simulink model "Feeder_IREQ_2012"  (Simulink 8.3)
settings: Solver=FixedStepDiscrete  StartTime=0.0  StopTime=100  FixedStep=50e-6  RelTol=1e-3
InitFcn:
  | Ts= 50e-6;
undefined symbols (not defined in the file): D11, Delta, DiscIntNeverNeededParam, Ion, kaimal_num, Lithium, u0
libraries: powerlib x62, powerlib_extras x49, simulink x14, simulink_extras x12, sps_avr x2, electricdrivelib x1
(part 2 of 5)

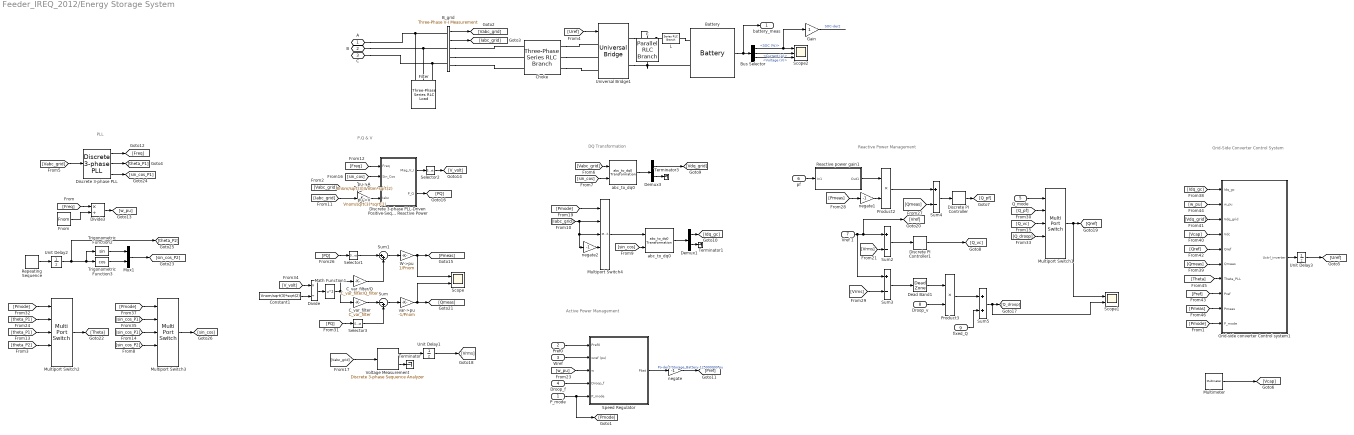
== system Feeder_IREQ_2012/Energy Storage System ==
  note: Grid-Side Converter
      | Control System
  note: DQ Transformation
  note: P,Q & V
  note: Reactive Power Management
  note: Active Power Management
  note: PLL
  P_mode : Inport
  Pref0 : Inport  Port=2
  Wref : Inport  Port=3
  Droop_f : Inport  Port=4
  Q_mode : Inport  Port=5
  "pf " : Inport  Port=6
  Vref 1 : Inport  Port=7
  Droop_v : Inport  Port=8
  fixed_Q : Inport  Port=9
  " C " : powerlib/Elements/Parallel RLC Branch  LConnTagsString=a  RConnTagsString=__new0  BranchType=C  Resistance=1  Inductance=1e-3  SetiL0=off  InitialCurrent=0  Capacitance=3000e-6  Setx0=on  InitialVoltage=Vbat  Measurements=Branch voltage
  B_grid : powerlib/Measurements/Three-Phase V-I Measurement  VoltageMeasurement=phase-to-ground  SetLabelV=off  LabelV=Vabc  Vpu=on  VpuLL=off  CurrentMeasurement=yes  SetLabelI=off  LabelI=Iabc  Ipu=on  Pbase=Pnom  Vbase=Vnom  OutputType=Complex  PhasorSimulation=off  PSBequivalent=0
  Battery : electricdrivelib/Extra Sources/Battery  BatType=Lithium-Ion  ShowDetailedParameters=off  NomV=Vbat  NomQ=Ebat/Vbat  SOC=SOC_initial  PresetModel=on  MaxQ=NaN  Dis_rate=NaN  Normal_OP=NaN  expZone="[NaN  NaN]"  Dis_Char=off  current=[1.5 3]  Units=Ampere-hour  Batt_Tr=10
  Bus Selector : BusSelector  OutputSignals=SOC (%),Current (A),Voltage (V)
  C_var_filter : Gain  Gain=C_var_filter  SaturateOnIntegerOverflow=on  OutDataTypeStr=Inherit: Same as input  ParamDataTypeStr=Inherit: Same as input
  C_var_filter/Q : Gain  Gain=C_var_filter/Q_filter  SaturateOnIntegerOverflow=on  OutDataTypeStr=Inherit: Same as input  ParamDataTypeStr=Inherit: Same as input
  "Choke " : powerlib/Elements/Three-Phase Series RLC Branch  LConnTagsString=A|B|C  RConnTagsString=A|B|C  BranchType=RL  Resistance=R_RL*Vnom^2/Pnom  Inductance=L_RL*Vnom^2/Pnom/(2*pi*Fnom)  Capacitance=[]  Measurements=None
  Constant1 : Constant  Value=Vnom/sqrt(3)*sqrt(2)
  Dead Band1 : DeadZone  LowerValue=-0.01  UpperValue=0.01  SaturateOnIntegerOverflow=on
  Demux1 : Demux  Outputs=[2 1]
  Demux3 : Demux  Outputs=[2 1]
  Discrete 3-phase PLL : powerlib_extras/Discrete  Control Blocks/Discrete 3-phase PLL  Fmin=0.75*Fnom  Par_Init=[-45 Fnom]  ParK=[60 1400 1]  Ts=Ts  AGC=off
  Discrete PI Controller : powerlib_extras/Discrete  Control Blocks/Discrete PI Controller  Kp=1  Ki=10  Par_Limits=[1 -1]  Init=0  Ts=-1
  Discrete PI Controller1 : powerlib_extras/Discrete  Control Blocks/Discrete PI Controller  Kp=2  Ki=20  Par_Limits=[1 -1]  Init=0  Ts=-1
  Discrete 3-phase PLL-Driven  Positive-Sequence Active & Reactive Power : Subsystem  mask(Discrete 3-phase PLL-Driven Positive-Sequence Active & Reactive Power){Finit=Fnom, Fmin=Fnom*45/60, Par_Vinit=[Vnom/sqrt(3)*sqrt(2) 30], Par_Iinit=[Pnom/sqrt(3)/Vnom*sqrt(2) -10], Ts=Ts}
      mask prompts: Finit "Initial frequency (Hz):"; Fmin "Minimum frequency (Hz):"; Par_Vinit "Voltage initial input: [ Mag  Phase(Degrees) ]"; Par_Iinit "Current initial input: [ Mag  Phase(Degrees) ]"; Ts "Sample time:"
      mask help:
      | This discrete block measures the 3-phase active power P and reactive power Q  associated with a periodic set of 3-phase voltages and currents which may contain harmonics. P and Q are calculated by evaluating the fundamental values (positive-sequence) of the input voltages and currents with a running window over one cycle of the specified frequency (port Freq).
      |  Input port "Sin_Cos" (a two-dimension signal) provides the reference frame required for the computation.
      |
      | input 1: must give the frequency of the fundamental (Hz)
      | Input 2: must contain a  [sin(wt)  cos(wt)] two dimension signal , where w is the rotation speed (rad/s) of the reference frame used for the computation..
      | input 3: Vectorized 3-phase  instantaneous voltage (Vabc)
      | input 4: Vectorized 3-phase instantaneous current (Iabc)
      |
      | Output 1: Vector [Mag_V Mag_I] of the fundamental values (Magnitude) of the voltage & current (peak values of the positive-sequence)
      | Output 2: 3-phase PQ measurement vector [P(W) Q (var)] evaluated at the specified frequency. Current flowing into an RL circuit will produce  positive active and reactive powers.
      |
      | For the first cycle of simulation, the outputs are held constant using the values specified by the parameters "Initial input".
      | he value of the parameter "Minimum frequency" is used to determine the buffer size of the "Variable Transport Delay" block found inside this subsystem.
      mask init:
      | power_initmask();
      settings: OpenFcn=power_openblockproxy();
  Divide : Product  Inputs=*/
  Divide3 : Product  Inputs=*/
  "Filter " : powerlib/Elements/Three-Phase Series RLC Load  LConnTagsString=A|B|C  Configuration=Y (grounded)  NominalVoltage=Vnom  NominalFrequency=Fnom  ActivePower=C_var_filter/Q_filter  InductivePower=0  CapacitivePower=C_var_filter  Measurements=None  LoadType=constant Z
  Fnom : Constant  Value=Fnom
  Gain : Gain
  Grid-side converter Control system1 : Subsystem
  L : powerlib/Elements/Series RLC Branch  LConnTagsString=__new0  RConnTagsString=__new0  BranchType=L  Resistance=1  Inductance=10e-6  SetiL0=off  InitialCurrent=0  Capacitance=1e-6  Setx0=off  InitialVoltage=0  Measurements=None
  Math Function1 : Math  Operator=square  SaturateOnIntegerOverflow=on
  Multimeter : powerlib/Measurements/Multimeter  PhasorSimulation=off  OutputType=Complex  sel=2  L=3  Gain=1  yselected={'Ub: Energy Storage System/ C '};  PSBOutputType=1  PSBequivalent=0  AxesSetting=[0,0.1,-100,100]  Display=0  SavedBlockNames=-11
  Multiport Switch{1..4} (4 alike) : MultiPortSwitch  Inputs=4  SaturateOnIntegerOverflow=on  InputSameDT=on
  Mux1 : Mux  Inputs=2
  Product2 : Product  RndMeth=Zero
  Product3 : Product  RndMeth=Zero
  Reactive power gain1 : Subsystem
  Repeating Sequence : simulink/Sources/Repeating Sequence  rep_seq_t=[0 1/60]  rep_seq_y=[0 2*pi]
  Scope : Scope  NumInputPorts=2
  Scope1 : Scope  NumInputPorts=2
  Scope2 : Scope  NumInputPorts=3
  Selector1 : Selector  InputPortWidth=2
  Selector2 : Selector  InputPortWidth=2
  Selector3 : Selector  InputPortWidth=2  Indices=2
  Speed Regulator : Subsystem  mask(Active Power Control){}
  Sum : Sum  Inputs=|-+
  Sum1 : Sum  Inputs=|++
  Sum2 : Sum  Inputs=+-  SaturateOnIntegerOverflow=on  InputSameDT=on  OutDataTypeStr=Inherit: Same as first input
  Sum3 : Sum  Inputs=+-  SaturateOnIntegerOverflow=on  InputSameDT=on  OutDataTypeStr=Inherit: Same as first input
  Sum4 : Sum  Inputs=+-  SaturateOnIntegerOverflow=on  InputSameDT=on  OutDataTypeStr=Inherit: Same as first input
  Sum5 : Sum  SaturateOnIntegerOverflow=on  InputSameDT=on  OutDataTypeStr=Inherit: Same as first input
  Terminator : Terminator
  Terminator1 : Terminator
  Terminator3 : Terminator
  Trigonometric Function2 : Trigonometry
  Trigonometric Function3 : Trigonometry  Operator=cos
  Unit Delay1 : UnitDelay  InitialCondition=1  SampleTime=Ts
  Unit Delay2 : UnitDelay  SampleTime=Ts
  Unit Delay3 : UnitDelay  SampleTime=Ts
  Universal Bridge1 : powerlib/Power Electronics/Universal Bridge  Arms=3  SnubberResistance=1e5  SnubberCapacitance=inf  Device=Average-model based VSC  Ron=1e-3  Lon=0  ForwardVoltages="[  0  0  ]"  ForwardVoltage=0  GTOparameters=[ 10e-6 , 20e-6 ]  IGBTparameters=[ 1e-6 , 2e-6 ]  Measurements=None  Measurements_2=None  converterType=Rectifier
  Voltage Measurement : powerlib_extras/Discrete Measurements/Discrete 3-phase Sequence Analyzer  Freq=60  n=1  seq=Positive  Par_Init=[1 0]  Ts=50e-6
  W->pu : Gain  Gain=1/Pnom  SaturateOnIntegerOverflow=on  OutDataTypeStr=Inherit: Same as input  ParamDataTypeStr=Inherit: Same as input
  abc_to_dq0 : powerlib_extras/Measurements/abc_to_dq0 Transformation
  "abc_to_dq0  " : powerlib_extras/Measurements/abc_to_dq0 Transformation
  negate : Gain  Gain=-1  SaturateOnIntegerOverflow=on  OutDataTypeStr=Inherit: Same as input  ParamDataTypeStr=Inherit: Same as input
  negate1 : Gain  Gain=-1  SaturateOnIntegerOverflow=on  OutDataTypeStr=Inherit: Same as input  ParamDataTypeStr=Inherit: Same as input
  negate2 : Gain  Gain=-1  SaturateOnIntegerOverflow=on  OutDataTypeStr=Inherit: Same as input  ParamDataTypeStr=Inherit: Same as input
  pu->A : Gain  Gain=Pnom/sqrt(3)/Vnom*sqrt(2)  SaturateOnIntegerOverflow=on  OutDataTypeStr=Inherit: Same as input  ParamDataTypeStr=Inherit: Same as input
  pu->V : Gain  Gain=Vnom/sqrt(3)*sqrt(2)  SaturateOnIntegerOverflow=on  OutDataTypeStr=Inherit: Same as input  ParamDataTypeStr=Inherit: Same as input
  "var->pu " : Gain  Gain=-1/Pnom  SaturateOnIntegerOverflow=on  OutDataTypeStr=Inherit: Same as input  ParamDataTypeStr=Inherit: Same as input
  A : PMIOPort  Port=1  Side=Right
  B : PMIOPort  Port=2  Side=Right
  C : PMIOPort  Port=3  Side=Right
  battery_meas : Outport
  wires:
  Grid-side converter Control system1/1(Uctrl_inverter) -> Unit Delay3/1
  Fnom/1 -> Divide3/2
  Divide3/1 -> [w_pu]
  [Freq] -> Divide3/1
  Demux1/2 -> Terminator1/1
  Demux3/2 -> Terminator3/1
  "abc_to_dq0  "/1 -> Demux1/1
  abc_to_dq0/1 -> Demux3/1
  [Vabc_grid] -> abc_to_dq0/1
  [sin_cos] -> abc_to_dq0/2
  [sin_cos] -> "abc_to_dq0  "/2
  B_grid/1 -> [Vabc_grid]
  B_grid/2 -> [Iabc_grid]
  Unit Delay3/1 -> [Uref]
  Selector2/1 -> [V_volt]
  Discrete 3-phase PLL-Driven  Positive-Sequence Active & Reactive Power/1(Mag_V_I) -> Selector2/1
  pu->V/1 -> Discrete 3-phase PLL-Driven  Positive-Sequence Active & Reactive Power/3(Vabc)
  [Freq] -> Discrete 3-phase PLL-Driven  Positive-Sequence Active & Reactive Power/1(Freq)
  [sin_cos] -> Discrete 3-phase PLL-Driven  Positive-Sequence Active & Reactive Power/2(Sin_Cos)
  pu->A/1 -> Discrete 3-phase PLL-Driven  Positive-Sequence Active & Reactive Power/4(Iabc)
  [Vabc_grid] -> pu->V/1
  [Iabc_grid] -> pu->A/1
  Discrete 3-phase PLL-Driven  Positive-Sequence Active & Reactive Power/2(P_Q) -> [PQ]
  "var->pu "/1 -> [Qmeas], Scope/2
  [PQ] -> Selector3/1
  W->pu/1 -> [Pmeas], Scope/1
  [PQ] -> Selector1/1
  [V_volt] -> Divide/1
  Constant1/1 -> Divide/2
  Divide/1 -> Math Function1/1
  Selector3/1 -> Sum/2
  Sum/1 -> "var->pu "/1
  Math Function1/1 -> C_var_filter/Q/1, C_var_filter/1
  Selector1/1 -> Sum1/1
  Sum1/1 -> W->pu/1
  [Uref] -> Universal Bridge1/1
  [Qmeas] -> Sum4/2
  Sum4/1 -> Discrete PI Controller/1
  [Pmeas] -> negate1/1
  Vref 1/1 -> [Vref], Sum2/1, Sum3/1
  [Vrms] -> Sum2/2
  Sum2/1 -> Discrete PI Controller1/1
  Reactive power gain1/1(Out1) -> Product2/1
  Product2/1 -> Sum4/1
  [Vrms] -> Sum3/2
  Sum3/1 -> Dead Band1/1
  Discrete PI Controller/1 -> [Q_pf]
  Dead Band1/1 -> Product3/1
  Droop_v/1 -> Product3/2
  Product3/1 -> Sum5/1
  Sum5/1 -> Scope1/2, [Q_droop]
  fixed_Q/1 -> Sum5/2
  [Q_pf] -> Multiport Switch1/2
  [Q_vc] -> Multiport Switch1/3
  [Q_droop] -> Multiport Switch1/4
  Q_mode/1 -> Multiport Switch1/1
  [Vabc_grid] -> Voltage Measurement/1
  Voltage Measurement/2 -> Terminator/1
  Voltage Measurement/1 -> Unit Delay1/1
  Unit Delay1/1 -> [Vrms]
  Pref0/1 -> Speed Regulator/1(Pref0)
  Wref/1 -> Speed Regulator/2(wref (pu))
  [w_pu] -> Speed Regulator/3(w)
  Droop_f/1 -> Speed Regulator/4(Droop_f)
  P_mode/1 -> Speed Regulator/5(P_mode), [Pmode]
  Speed Regulator/1(Pbat) -> negate/1
  Multiport Switch1/1 -> Scope1/1, [Qref]
  negate1/1 -> Product2/2
  "pf "/1 -> Reactive power gain1/1(In1)
  Multimeter/1 -> [Vcap]
  Trigonometric Function3/1 -> Mux1/2
  Trigonometric Function2/1 -> Mux1/1
  Unit Delay2/1 -> [theta_P2], Trigonometric Function2/1, Trigonometric Function3/1
  [Vabc_grid] -> Discrete 3-phase PLL/1
  Discrete 3-phase PLL/1 -> [Freq]
  Discrete 3-phase PLL/2 -> [theta_P1]
  Discrete 3-phase PLL/3 -> [sin_cos_P1]
  Mux1/1 -> [sin_cos_P2]
  [theta_P1] -> Multiport Switch2/2
  [Pmode] -> Multiport Switch2/1
  [sin_cos_P1] -> Multiport Switch3/2
  [Pmode] -> Multiport Switch3/1
  Multiport Switch2/1 -> [Theta]
  Multiport Switch3/1 -> [sin_cos]
  Discrete PI Controller1/1 -> [Q_vc]
  Repeating Sequence/1 -> Unit Delay2/1
  Demux3/1 -> [Vdq_grid]
  Demux1/1 -> [Idq_gc]
  [Idq_gc] -> Grid-side converter Control system1/1(Idq_gc)
  [w_pu] -> Grid-side converter Control system1/2(w_pu)
  [Vdq_grid] -> Grid-side converter Control system1/3(Vdq_grid)
  [Vcap] -> Grid-side converter Control system1/4(Vdc)
  [Qref] -> Grid-side converter Control system1/5(Qref)
  [Qmeas] -> Grid-side converter Control system1/6(Qmeas)
  [Theta] -> Grid-side converter Control system1/7(Theta_PLL)
  [Pref] -> Grid-side converter Control system1/8(Pref)
  [Pmeas] -> Grid-side converter Control system1/9(Pmeas)
  [Pmode] -> Grid-side converter Control system1/10(P_mode)
  [theta_P2] -> Multiport Switch2/4
  [sin_cos_P2] -> Multiport Switch3/4
  negate/1 -> [Pref]  "Po-der2-Storage_Battery-125000000-pu"
  [Pmode] -> Multiport Switch4/1
  [Iabc_grid] -> negate2/1, Multiport Switch4/3, Multiport Switch4/2
  negate2/1 -> Multiport Switch4/4
  Multiport Switch4/1 -> "abc_to_dq0  "/1
  C_var_filter/Q/1 -> Sum1/2
  C_var_filter/1 -> Sum/1
  [theta_P1] -> Multiport Switch2/3
  [sin_cos_P1] -> Multiport Switch3/3
  Battery/1 -> battery_meas/1, Bus Selector/1
  Bus Selector/2 -> Scope2/2  "<Current (A)>"
  Bus Selector/1 -> Gain/1, Scope2/1  "<SOC (%)>"
  Bus Selector/3 -> Scope2/3  "<Voltage (V)>"
  Gain/1 -> ?  "SOC-der2"
  connections:
  B_grid/RConn1 -- "Choke "/LConn1
  B_grid/RConn2 -- "Choke "/LConn2
  B_grid/RConn3 -- "Choke "/LConn3
  "Choke "/RConn1 -- Universal Bridge1/LConn1
  "Choke "/RConn2 -- Universal Bridge1/LConn2
  "Choke "/RConn3 -- Universal Bridge1/LConn3
  C/RConn1 -- "Filter "/LConn3 -- B_grid/LConn3
  B/RConn1 -- "Filter "/LConn2 -- B_grid/LConn2
  A/RConn1 -- B_grid/LConn1 -- "Filter "/LConn1
  L/LConn1 -- Universal Bridge1/RConn1 -- " C "/LConn1
  L/RConn1 -- Battery/LConn1
  Universal Bridge1/RConn2 -- " C "/RConn1 -- Battery/LConn2

== system Feeder_IREQ_2012/Kaimal Wind Speed Profile ==
  Band-Limited White Noise : simulink/Sources/Band-Limited White Noise  Cov=[1]  Ts=.05  seed=[53489]
  Constant4 : Constant  Value=Mean_wind
  Constant6 : Constant  Value=trans/sqrt(2)
  Product : Product  SampleTime=.05  RndMeth=Zero
  Rate Transition : RateTransition
  Sum1 : Sum  SampleTime=.05  SaturateOnIntegerOverflow=on  InputSameDT=on  OutDataTypeStr=Inherit: Same as first input
  Transfer Fcn Direct Form II : simulink/Additional Math & Discrete/Additional Discrete/Transfer Fcn Direct Form II  NumCoefVec=[kaimal_num]  DenCoefVec=[kaimal_den(2:end)]  vinit=0.0  DoSatur=off
  Unit Delay : UnitDelay  SampleTime=.05
  wind profile : Outport  InitialOutput=[u0]
  wires:
  Product/1 -> Sum1/2
  Constant6/1 -> Product/2
  Sum1/1 -> [wind], Rate Transition/1
  Constant4/1 -> Sum1/1
  Band-Limited White Noise/1 -> Unit Delay/1
  Transfer Fcn Direct Form II/1 -> Product/1
  Unit Delay/1 -> Transfer Fcn Direct Form II/1
  Rate Transition/1 -> wind profile/1

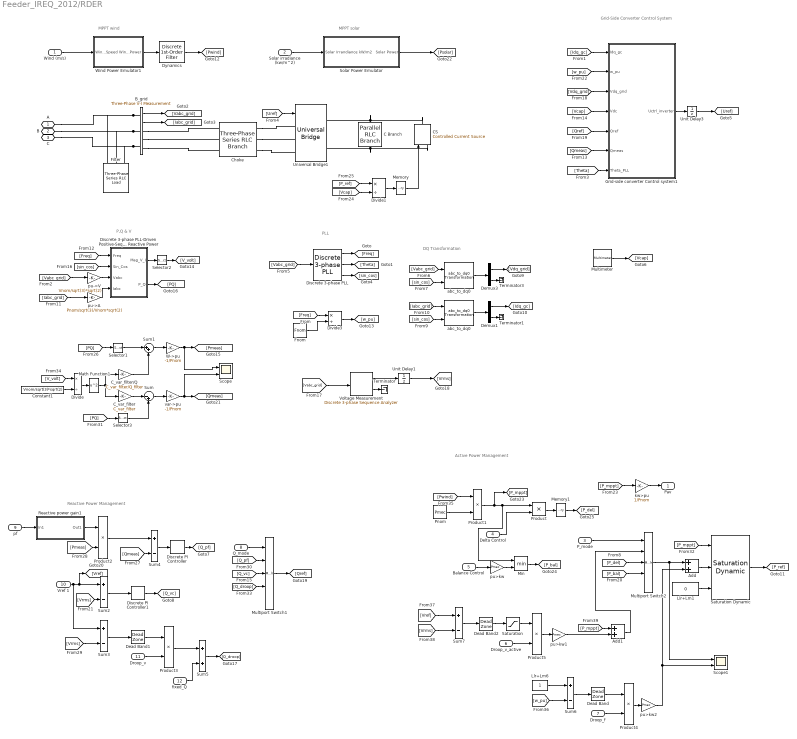
== system Feeder_IREQ_2012/RDER ==
  note: Grid-Side Converter
      | Control System
  note: PLL
  note: DQ Transformation
  note: P,Q & V
  note: Reactive Power Management
  note: Active Power Management
  note: MPPT wind
  note: MPPT solar
  "Wind (m/s) " : Inport
  Solar irradiance (kw/m^2) : Inport  Port=2
  P_mode : Inport  Port=3
  Delta Control : Inport  Port=4
  Balance Control : Inport  Port=5
  Droop_v_active : Inport  Port=6
  Droop_f : Inport  Port=7
  Q_mode : Inport  Port=8
  "pf " : Inport  Port=9
  Vref 1 : Inport  Port=10
  Droop_v : Inport  Port=11
  fixed_Q : Inport  Port=12
  " C Branch" : powerlib/Elements/Parallel RLC Branch  LConnTagsString=a  RConnTagsString=__new0  BranchType=C  Resistance=1  Inductance=1e-3  SetiL0=off  InitialCurrent=0  Capacitance=2000e-6  Setx0=on  InitialVoltage=Vdc_nom  Measurements=Branch voltage
  Add : Sum
  Add1 : Sum
  B_grid : powerlib/Measurements/Three-Phase V-I Measurement  VoltageMeasurement=phase-to-ground  SetLabelV=off  LabelV=Vabc  Vpu=on  VpuLL=off  CurrentMeasurement=yes  SetLabelI=off  LabelI=Iabc  Ipu=on  Pbase=Pnom  Vbase=Vnom  OutputType=Complex  PhasorSimulation=off  PSBequivalent=0
  CS : powerlib/Electrical Sources/Controlled Current Source  Initialize=on  Source_Type=AC  Amplitude=0  Phase=0  Frequency=0  Measurements=None
  C_var_filter : Gain  Gain=C_var_filter  SaturateOnIntegerOverflow=on  OutDataTypeStr=Inherit: Same as input  ParamDataTypeStr=Inherit: Same as input
  C_var_filter/Q : Gain  Gain=C_var_filter/Q_filter  SaturateOnIntegerOverflow=on  OutDataTypeStr=Inherit: Same as input  ParamDataTypeStr=Inherit: Same as input
  "Choke " : powerlib/Elements/Three-Phase Series RLC Branch  LConnTagsString=A|B|C  RConnTagsString=A|B|C  BranchType=RL  Resistance=R_RL*Vnom^2/Pnom  Inductance=L_RL*Vnom^2/Pnom/(2*pi*Fnom)  Capacitance=[]  Measurements=None
  Constant1 : Constant  Value=Vnom/sqrt(3)*sqrt(2)
  Dead Band : DeadZone  LowerValue=-0.001  UpperValue=0.001  SaturateOnIntegerOverflow=on
  Dead Band1 : DeadZone  LowerValue=-0.01  UpperValue=0.01  SaturateOnIntegerOverflow=on
  Dead Band2 : DeadZone  LowerValue=-0.01  UpperValue=0.01  SaturateOnIntegerOverflow=on
  Demux1 : Demux  Outputs=[2 1]
  Demux3 : Demux  Outputs=[2 1]
  Discrete 3-phase PLL : powerlib_extras/Discrete  Control Blocks/Discrete 3-phase PLL  Fmin=0.75*Fnom  Par_Init=[-45 Fnom]  ParK=[60 1400 1]  Ts=Ts  AGC=off
  Discrete PI Controller : powerlib_extras/Discrete  Control Blocks/Discrete PI Controller  Kp=1  Ki=10  Par_Limits=[1 -1]  Init=0  Ts=-1
  Discrete PI Controller1 : powerlib_extras/Discrete  Control Blocks/Discrete PI Controller  Kp=1  Ki=10  Par_Limits=[1 -1]  Init=0  Ts=-1
  Discrete 3-phase PLL-Driven  Positive-Sequence Active & Reactive Power : Subsystem  mask(Discrete 3-phase PLL-Driven Positive-Sequence Active & Reactive Power){Finit=Fnom, Fmin=Fnom*45/60, Par_Vinit=[Vnom/sqrt(3)*sqrt(2) 30], Par_Iinit=[Pnom/sqrt(3)/Vnom*sqrt(2) -10], Ts=Ts}
      mask prompts: Finit "Initial frequency (Hz):"; Fmin "Minimum frequency (Hz):"; Par_Vinit "Voltage initial input: [ Mag  Phase(Degrees) ]"; Par_Iinit "Current initial input: [ Mag  Phase(Degrees) ]"; Ts "Sample time:"
      mask help:
      | This discrete block measures the 3-phase active power P and reactive power Q  associated with a periodic set of 3-phase voltages and currents which may contain harmonics. P and Q are calculated by evaluating the fundamental values (positive-sequence) of the input voltages and currents with a running window over one cycle of the specified frequency (port Freq).
      |  Input port "Sin_Cos" (a two-dimension signal) provides the reference frame required for the computation.
      |
      | input 1: must give the frequency of the fundamental (Hz)
      | Input 2: must contain a  [sin(wt)  cos(wt)] two dimension signal , where w is the rotation speed (rad/s) of the reference frame used for the computation..
      | input 3: Vectorized 3-phase  instantaneous voltage (Vabc)
      | input 4: Vectorized 3-phase instantaneous current (Iabc)
      |
      | Output 1: Vector [Mag_V Mag_I] of the fundamental values (Magnitude) of the voltage & current (peak values of the positive-sequence)
      | Output 2: 3-phase PQ measurement vector [P(W) Q (var)] evaluated at the specified frequency. Current flowing into an RL circuit will produce  positive active and reactive powers.
      |
      | For the first cycle of simulation, the outputs are held constant using the values specified by the parameters "Initial input".
      | he value of the parameter "Minimum frequency" is used to determine the buffer size of the "Variable Transport Delay" block found inside this subsystem.
      mask init:
      | power_initmask();
      settings: OpenFcn=power_openblockproxy();
  Divide : Product  Inputs=*/
  Divide1 : Product  Inputs=*/
  Divide3 : Product  Inputs=*/
  Dynamics : powerlib_extras/Discrete  Control Blocks/Discrete 1st-Order Filter  FilterType=Lowpass  Tc=1/3  Ts=50e-6  Initialize=off  Vac_Init=[0.8 -25 60]  Vdc_Init=1  PlotResponse=off  param1=[1 500 0.1]
  "Filter " : powerlib/Elements/Three-Phase Series RLC Load  LConnTagsString=A|B|C  Configuration=Y (grounded)  NominalVoltage=Vnom  NominalFrequency=Fnom  ActivePower=C_var_filter/Q_filter  InductivePower=0  CapacitivePower=C_var_filter  Measurements=None  LoadType=constant Z
  Fnom : Constant  Value=Fnom
  Grid-side converter Control system1 : Subsystem
  Llr+Lm1 : Constant  Value=0
  Llr+Lm6 : Constant
  Math Function1 : Math  Operator=square  SaturateOnIntegerOverflow=on
  Memory : Memory  X0=100
  Memory1 : Memory  X0=.8
  Min : MinMax  Inputs=2
  Multimeter : powerlib/Measurements/Multimeter  PhasorSimulation=off  OutputType=Complex  sel=3  L=3  Gain=1  yselected={'Ub: RDER/ C Branch'};  PSBOutputType=1  PSBequivalent=0  AxesSetting=[0,0.1,-100,100]  Display=0  SavedBlockNames=-11
  Multiport Switch1 : MultiPortSwitch  Inputs=4  SaturateOnIntegerOverflow=on  InputSameDT=on
  Multiport Switch2 : MultiPortSwitch  Inputs=4  SaturateOnIntegerOverflow=on  InputSameDT=on
  Pnom : Constant  Value=Pmec
  Product{,1..5} (6 alike) : Product  RndMeth=Zero
  Reactive power gain1 : Subsystem
  Saturation : Saturate  UpperLimit=0  LowerLimit=-1
  Saturation Dynamic : simulink/Discontinuities/Saturation Dynamic  OutMin=[]  OutMax=[]  OutDataTypeStr=Inherit: Same as second input  OutDataType=fixdt(1, 16)  OutScaling=2^-10  DoSatur=off
  Scope : Scope  NumInputPorts=2
  Scope1 : Scope  NumInputPorts=2
  Selector1 : Selector  InputPortWidth=2
  Selector2 : Selector  InputPortWidth=2
  Selector3 : Selector  InputPortWidth=2  Indices=2
  Solar Power Emulator : Subsystem
  Sum : Sum  Inputs=|-+
  Sum1 : Sum  Inputs=|++
  Sum{2..4,6..7} (5 alike) : Sum  Inputs=+-  SaturateOnIntegerOverflow=on  InputSameDT=on  OutDataTypeStr=Inherit: Same as first input
  Sum5 : Sum  SaturateOnIntegerOverflow=on  InputSameDT=on  OutDataTypeStr=Inherit: Same as first input
  Terminator : Terminator
  Terminator1 : Terminator
  Terminator3 : Terminator
  Unit Delay1 : UnitDelay  InitialCondition=1  SampleTime=Ts
  Unit Delay3 : UnitDelay  SampleTime=Ts
  Universal Bridge1 : powerlib/Power Electronics/Universal Bridge  Arms=3  SnubberResistance=1e5  SnubberCapacitance=inf  Device=Average-model based VSC  Ron=1e-3  Lon=0  ForwardVoltages="[  0  0  ]"  ForwardVoltage=0  GTOparameters=[ 10e-6 , 20e-6 ]  IGBTparameters=[ 1e-6 , 2e-6 ]  Measurements=None  Measurements_2=None  converterType=Rectifier
  Voltage Measurement : powerlib_extras/Discrete Measurements/Discrete 3-phase Sequence Analyzer  Freq=60  n=1  seq=Positive  Par_Init=[1 0]  Ts=50e-6
  W->pu : Gain  Gain=-1/Pnom  SaturateOnIntegerOverflow=on  OutDataTypeStr=Inherit: Same as input  ParamDataTypeStr=Inherit: Same as input
  Wind Power Emulator1 : Subsystem
  abc_to_dq0 : powerlib_extras/Measurements/abc_to_dq0 Transformation
  "abc_to_dq0  " : powerlib_extras/Measurements/abc_to_dq0 Transformation
  kw>pu : Gain  Gain=1/Pnom
  pu->A : Gain  Gain=Pnom/sqrt(3)/Vnom*sqrt(2)  SaturateOnIntegerOverflow=on  OutDataTypeStr=Inherit: Same as input  ParamDataTypeStr=Inherit: Same as input
  pu->V : Gain  Gain=Vnom/sqrt(3)*sqrt(2)  SaturateOnIntegerOverflow=on  OutDataTypeStr=Inherit: Same as input  ParamDataTypeStr=Inherit: Same as input
  pu>kw : Gain  Gain=Pmec
  pu>kw1 : Gain  Gain=Pmec
  pu>kw2 : Gain  Gain=Pmec
  "var->pu " : Gain  Gain=-1/Pnom  SaturateOnIntegerOverflow=on  OutDataTypeStr=Inherit: Same as input  ParamDataTypeStr=Inherit: Same as input
  A : PMIOPort  Port=1  Side=Right
  B : PMIOPort  Port=2  Side=Right
  C : PMIOPort  Port=3  Side=Right
  Pav : Outport
  wires:
  [Idq_gc] -> Grid-side converter Control system1/1(Idq_gc)
  [w_pu] -> Grid-side converter Control system1/2(w_pu)
  [Vdq_grid] -> Grid-side converter Control system1/3(Vdq_grid)
  [Vcap] -> Grid-side converter Control system1/4(Vdc)
  [Qmeas] -> Grid-side converter Control system1/6(Qmeas)
  Grid-side converter Control system1/1(Uctrl_inverter) -> Unit Delay3/1
  Discrete 3-phase PLL/1 -> [Freq]
  Fnom/1 -> Divide3/2
  Divide3/1 -> [w_pu]
  Discrete 3-phase PLL/3 -> [sin_cos]
  [Freq] -> Divide3/1
  Discrete 3-phase PLL/2 -> [Theta]
  [Vabc_grid] -> Discrete 3-phase PLL/1
  Demux1/2 -> Terminator1/1
  Demux3/1 -> [Vdq_grid]
  Demux3/2 -> Terminator3/1
  "abc_to_dq0  "/1 -> Demux1/1
  abc_to_dq0/1 -> Demux3/1
  [Vabc_grid] -> abc_to_dq0/1
  [sin_cos] -> abc_to_dq0/2
  [sin_cos] -> "abc_to_dq0  "/2
  [Iabc_grid] -> "abc_to_dq0  "/1
  Demux1/1 -> [Idq_gc]
  B_grid/1 -> [Vabc_grid]
  B_grid/2 -> [Iabc_grid]
  Unit Delay3/1 -> [Uref]
  Selector2/1 -> [V_volt]
  Discrete 3-phase PLL-Driven  Positive-Sequence Active & Reactive Power/1(Mag_V_I) -> Selector2/1
  pu->V/1 -> Discrete 3-phase PLL-Driven  Positive-Sequence Active & Reactive Power/3(Vabc)
  [Freq] -> Discrete 3-phase PLL-Driven  Positive-Sequence Active & Reactive Power/1(Freq)
  [sin_cos] -> Discrete 3-phase PLL-Driven  Positive-Sequence Active & Reactive Power/2(Sin_Cos)
  pu->A/1 -> Discrete 3-phase PLL-Driven  Positive-Sequence Active & Reactive Power/4(Iabc)
  [Vabc_grid] -> pu->V/1
  [Iabc_grid] -> pu->A/1
  Discrete 3-phase PLL-Driven  Positive-Sequence Active & Reactive Power/2(P_Q) -> [PQ]
  "var->pu "/1 -> [Qmeas], Scope/2
  [PQ] -> Selector3/1
  W->pu/1 -> [Pmeas], Scope/1
  [PQ] -> Selector1/1
  [V_volt] -> Divide/1
  Constant1/1 -> Divide/2
  Divide/1 -> Math Function1/1
  Selector3/1 -> Sum/2
  Sum/1 -> "var->pu "/1
  Math Function1/1 -> C_var_filter/Q/1, C_var_filter/1
  Selector1/1 -> Sum1/1
  Sum1/1 -> W->pu/1
  [Uref] -> Universal Bridge1/1
  Multimeter/1 -> [Vcap]
  [Qmeas] -> Sum4/2
  Sum4/1 -> Discrete PI Controller/1
  [Pmeas] -> Product2/2
  Vref 1/1 -> [Vref], Sum2/1, Sum3/1
  [Vrms] -> Sum2/2
  Sum2/1 -> Discrete PI Controller1/1
  Reactive power gain1/1(Out1) -> Product2/1
  Product2/1 -> Sum4/1
  [Vrms] -> Sum3/2
  Sum3/1 -> Dead Band1/1
  Discrete PI Controller/1 -> [Q_pf]
  Discrete PI Controller1/1 -> [Q_vc]
  Dead Band1/1 -> Product3/1
  Droop_v/1 -> Product3/2
  Product3/1 -> Sum5/1
  Sum5/1 -> [Q_droop]
  fixed_Q/1 -> Sum5/2
  [Q_pf] -> Multiport Switch1/2
  [Q_vc] -> Multiport Switch1/3
  [Q_droop] -> Multiport Switch1/4
  Q_mode/1 -> Multiport Switch1/1
  [Vabc_grid] -> Voltage Measurement/1
  Voltage Measurement/2 -> Terminator/1
  Voltage Measurement/1 -> Unit Delay1/1
  Unit Delay1/1 -> [Vrms]
  Divide1/1 -> Memory/1
  [Vcap] -> Divide1/2
  [P_ref] -> Divide1/1
  Memory/1 -> CS/1
  "Wind (m/s) "/1 -> Wind Power Emulator1/1(Wind Speed)
  [Theta] -> Grid-side converter Control system1/7(Theta_PLL)
  [Qref] -> Grid-side converter Control system1/5(Qref)
  Pnom/1 -> Product1/2
  [Pwind] -> Product1/1
  Product1/1 -> [P_mppt], Min/1, Product/1
  Delta Control/1 -> Product/2
  kw>pu/1 -> Pav/1
  Balance Control/1 -> pu>kw/1
  pu>kw/1 -> Min/2
  Min/1 -> [P_bal]
  Product/1 -> Memory1/1
  Add1/1 -> Multiport Switch2/2
  [P_del] -> Multiport Switch2/3
  [P_bal] -> Multiport Switch2/4
  P_mode/1 -> Multiport Switch2/1
  Multiport Switch2/1 -> Scope1/1, Add/1
  Llr+Lm6/1 -> Sum6/1
  [w_pu] -> Sum6/2
  Sum6/1 -> Dead Band/1
  Dead Band/1 -> Product4/1
  Add/1 -> Saturation Dynamic/2
  Saturation Dynamic/1 -> [P_ref]
  [P_mppt] -> Saturation Dynamic/1
  Llr+Lm1/1 -> Saturation Dynamic/3
  Droop_f/1 -> Product4/2
  Product4/1 -> pu>kw2/1
  [Vref] -> Sum7/1
  [Vrms] -> Sum7/2
  Sum7/1 -> Dead Band2/1
  Dead Band2/1 -> Saturation/1
  Droop_v_active/1 -> Product5/2
  Product5/1 -> pu>kw1/1
  [P_mppt] -> Add1/1
  Saturation/1 -> Product5/1
  pu>kw1/1 -> Add1/2
  [P_mppt] -> kw>pu/1
  Dynamics/1 -> [Pwind]
  Solar Power Emulator/1(Solar Power) -> [Psolar]
  Wind Power Emulator1/1(Wind Power) -> Dynamics/1
  Solar irradiance (kw/m^2)/1 -> Solar Power Emulator/1(Solar Irrandiance kW/m2)
  C_var_filter/Q/1 -> Sum1/2
  C_var_filter/1 -> Sum/1
  Multiport Switch1/1 -> [Qref]
  "pf "/1 -> Reactive power gain1/1(In1)
  pu>kw2/1 -> Scope1/2, Add/2
  Memory1/1 -> [P_del]
  connections:
  B_grid/RConn1 -- "Choke "/LConn1
  B_grid/RConn2 -- "Choke "/LConn2
  B_grid/RConn3 -- "Choke "/LConn3
  "Choke "/RConn1 -- Universal Bridge1/LConn1
  "Choke "/RConn2 -- Universal Bridge1/LConn2
  "Choke "/RConn3 -- Universal Bridge1/LConn3
  B_grid/LConn3 -- C/RConn1 -- "Filter "/LConn3
  B_grid/LConn2 -- B/RConn1 -- "Filter "/LConn2
  B_grid/LConn1 -- A/RConn1 -- "Filter "/LConn1
  CS/RConn1 -- " C Branch"/LConn1 -- Universal Bridge1/RConn1
  CS/LConn1 -- " C Branch"/RConn1 -- Universal Bridge1/RConn2

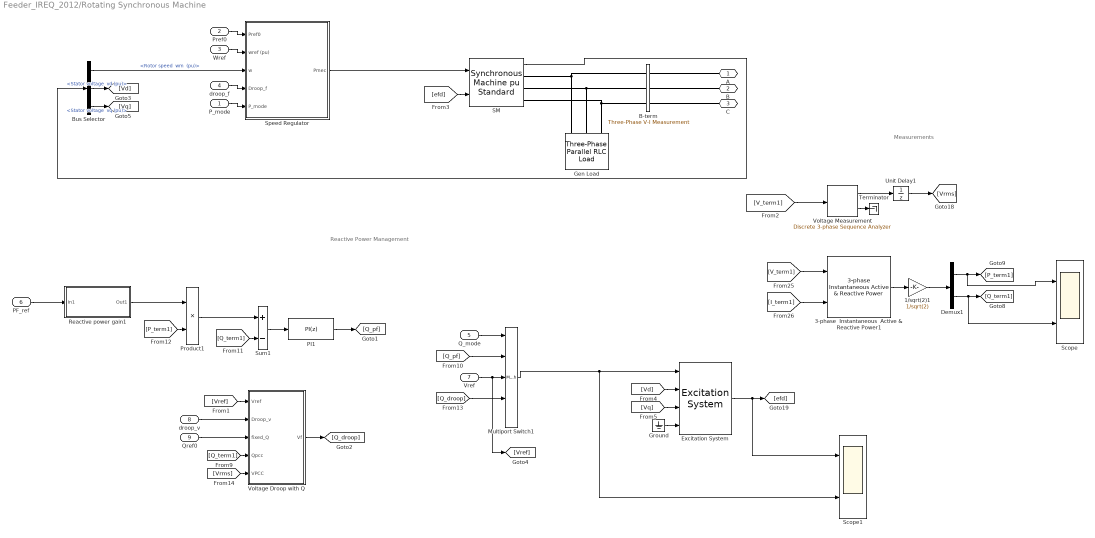
== system Feeder_IREQ_2012/Rotating Synchronous Machine ==
  note: Reactive Power Management
  note: Measurements
  P_mode : Inport
  Pref0 : Inport  Port=2
  Wref : Inport  Port=3
  droop_f : Inport  Port=4
  Q_mode : Inport  Port=5
  PF_ref : Inport  Port=6
  Vref : Inport  Port=7
  droop_v : Inport  Port=8
  Qref0 : Inport  Port=9
  1/sqrt(2)1 : Gain  Gain=1/sqrt(2)
  3-phase  Instantaneous  Active & Reactive Power1 : powerlib_extras/Measurements/3-phase  Instantaneous  Active & Reactive Power
  B-term : powerlib/Measurements/Three-Phase V-I Measurement  VoltageMeasurement=phase-to-ground  SetLabelV=on  LabelV=V_term1  Vpu=on  VpuLL=off  CurrentMeasurement=yes  SetLabelI=on  LabelI=I_term1  Ipu=on  Pbase=Pnom  Vbase=600  OutputType=Complex  PhasorSimulation=off  PSBequivalent=0
  Bus Selector : BusSelector  OutputSignals="Mechanical.Rotor speed  wm  (pu),dq0 components.Stator voltage  vd (pu),dq0 components.Stator voltage  vq (pu)"
  Demux1 : Demux  Outputs=2
  "Excitation System " : sps_avr/Excitation System  tr=20e-3  reg=[ 300, 0.001 ]  exc=[ 1, 0 ]  tgr=[ 0, 0 ]  damp=[ 0.001, 0.1 ]  sat=[ 0, 0 ]  lim=[ -11.5, 11.5, 0 ]  v0="[1.0  1.28]"
  Gen Load : powerlib/Elements/Three-Phase Parallel RLC Load  LConnTagsString=A|B|C  Configuration=Y (grounded)  NominalVoltage=600  NominalFrequency=60  ActivePower=5e3  InductivePower=0  CapacitivePower=0  Measurements=None  LoadType=constant Z
  Ground : Ground
  Multiport Switch1 : MultiPortSwitch  Inputs=4  SaturateOnIntegerOverflow=on  InputSameDT=on
  PI1 : simulink/Continuous/PID Controller  Controller=PI  TimeDomain=Discrete-time  SampleTime=-1  IntegratorMethod=Forward Euler  FilterMethod=Forward Euler  Form=Parallel  P=1  I=20  D=-14.7932376623781  N=587.187356380874  InitialConditionSource=internal  InitialConditionForIntegrator=0  InitialConditionForFilter=0  ExternalReset=none  LimitOutput=on  UpperSaturationLimit=1.05  LowerSaturationLimit=.95  LinearizeAsGain=off  AntiWindupMode=back-calculation  Kb=1  TrackingMode=off  Kt=1  PParamMin=[]  PParamMax=[]  IParamMin=[]  IParamMax=[]  DParamMin=[]  DParamMax=[]  NParamMin=[]  NParamMax=[]  KbParamMin=[]  KbParamMax=[]  KtParamMin=[]  KtParamMax=[]  POutMin=[]  POutMax=[]  IOutMin=[]  IOutMax=[]  DOutMin=[]  DOutMax=[]  NOutMin=[]  NOutMax=[]  KbOutMin=[]  KbOutMax=[]  KtOutMin=[]  KtOutMax=[]  IntegratorOutMin=[]  IntegratorOutMax=[]  FilterOutMin=[]  FilterOutMax=[]  SumOutMin=[]  SumOutMax=[]  SumI1OutMin=[]  SumI1OutMax=[]  SumI2OutMin=[]  SumI2OutMax=[]  SumI3OutMin=[]  SumI3OutMax=[]  SumDOutMin=[]  SumDOutMax=[]  SaturationOutMin=[]  SaturationOutMax=[]  IntegratorContinuousStateAttributes=''  IntegratorStateMustResolveToSignalObject=off  IntegratorRTWStateStorageClass=Auto  FilterContinuousStateAttributes=''  FilterStateMustResolveToSignalObject=off  FilterRTWStateStorageClass=Auto
  Product1 : Product  RndMeth=Zero
  Reactive power gain1 : Subsystem
  SM : powerlib/Machines/Synchronous Machine pu Standard  PresetModel=No  MechanicalLoad=Mechanical power Pm  ShowDetailedParameters=on  RotorType=Round  Units=per unit standard parameters  MeasurementBus=off  NominalParameters="[ Pnom  600   60]"  Reactances1=[ 1.81, 0.3, 0.23, 1.76, 0.65, 0.25, 0.15 ]  Reactances2="[ 1.305, 0.296, 0.252, 0.474,  0.243,  0.18 ]"  dAxisTimeConstants=Open-circuit  qAxisTimeConstants=Short-circuit  TimeConstants1="[ 4.4849  0.0681  0.1  ]"  TimeConstants2=[ 8.0, 0.03, 1.0, 0.07 ]  TimeConstants3=[ 3, 0.05, 0.05 ]  TimeConstants4=[ 8.0, 0.03, 0.3371, 0.0295 ]  TimeConstants5=[ 1.01, 0.053, 0.1 ]  TimeConstants6=[ 1.3201, 0.023, 1.0, 0.07 ]  TimeConstants7=[0.012 0.003 0.003]  TimeConstants8=[ 1.3201, 0.0231, 0.3371, 0.0295 ]  StatorResistance=0.003  Mechanical=[ 1.2 0 4 ]  PolePairs=4  InitialConditions="[ 0  0  0  0  0  0  0  0  1 ]"  SetSaturation=off  Saturation=[0.6404,0.7127,0.8441,0.9214,0.9956,1.082,1.19,1.316,1.457;0.7,0.7698,0.8872,0.9466,0.9969,1.046,1.1,1.151,1.201]  LoadFlowParameters=[1,0,0,0,0]  TsPowergui=0  TsBlock=-1  IterativeModel=Trapezoidal non iterative  BusType=PV  Pref=0  Qref=0  Qmin=-inf  Qmax=inf  PLF=0  QLF=0
  Scope : Scope  NumInputPorts=2
  Scope1 : Scope  NumInputPorts=2
  Speed Regulator : Subsystem  mask(Diesel Engine & Governor){Tr=[0.01 0.02 0.05], Ta=[0.25 0.009 0.0384], Tlim=[0.0  1], Td=0.024, Pm0=0.25, K=40, Ts=Ts}
      mask prompts: Tr "Regulator time constants [T1 T2 ] (s) :"; Ta "Actuator time constants [T3 T4 T5] (s) :"; Tlim "Torque limits [Tmin Tmax] (pu) :"; Td "Engine time delay Td (s) :"; Pm0 "Initial value of mechanical power  Pm0 (pu) :"; K "Regulator gain K:"; Ts "Sample time"
      mask help:
      | Diesel engine and governor system. The input 1 is the measured speed, in rad/s. The input 2 is the reference speed, in pu. The output is the mechanical power.
      |
      | Controller transfer function:
      | Hc=K.(1+T1.s)/(1+T2.s)
      |
      | Throttle actuator transfer function :
      | Ha= (1+T3.s) / [ (s (1+T4.s)(1+T5.s) ]
      |
      | Motor :
      | Time delay Td
      | Inertia and viscous friction are modeled in the Synchronous generator.
      |
      | The base power used to specify the initial mechanical power (Pm0 in pu) is the nominal power of the driven generator
  Sum1 : Sum  Inputs=+-  SaturateOnIntegerOverflow=on  InputSameDT=on  OutDataTypeStr=Inherit: Same as first input
  Terminator : Terminator
  Unit Delay1 : UnitDelay  InitialCondition=1  SampleTime=-1
  Voltage Measurement : powerlib_extras/Discrete Measurements/Discrete 3-phase Sequence Analyzer  Freq=60  n=1  seq=Positive  Par_Init=[1 0]  Ts=50e-6
  Voltage Droop with Q : Subsystem
  A : PMIOPort  Port=1  Side=Right
  B : PMIOPort  Port=2  Side=Right
  C : PMIOPort  Port=3  Side=Right
  wires:
  Qref0/1 -> Voltage Droop with Q/3(fixed_Q)
  Voltage Droop with Q/1(Vf) -> [Q_droop]
  [Q_term1] -> Voltage Droop with Q/4(Qpcc)
  Q_mode/1 -> Multiport Switch1/1
  [P_term1] -> Product1/2
  Bus Selector/1 -> Speed Regulator/3(w)  "<Rotor speed  wm  (pu)>"
  Pref0/1 -> Speed Regulator/1(Pref0)
  SM/1 -> Bus Selector/1
  [Vrms] -> Voltage Droop with Q/5(VPCC)
  [Q_droop] -> Multiport Switch1/4
  [Q_pf] -> Multiport Switch1/2
  Vref/1 -> [Vref], Multiport Switch1/3
  PI1/1 -> [Q_pf]
  Reactive power gain1/1(Out1) -> Product1/1
  droop_v/1 -> Voltage Droop with Q/2(Droop_v)
  Sum1/1 -> PI1/1
  [Q_term1] -> Sum1/2
  [efd] -> SM/2
  Product1/1 -> Sum1/1
  PF_ref/1 -> Reactive power gain1/1(In1)
  Wref/1 -> Speed Regulator/2(wref (pu))
  droop_f/1 -> Speed Regulator/4(Droop_f)
  [Vref] -> Voltage Droop with Q/1(Vref)
  P_mode/1 -> Speed Regulator/5(P_mode)
  Voltage Measurement/2 -> Terminator/1
  Voltage Measurement/1 -> Unit Delay1/1
  Unit Delay1/1 -> [Vrms]
  [V_term1] -> Voltage Measurement/1
  [V_term1] -> 3-phase  Instantaneous  Active & Reactive Power1/1
  [I_term1] -> 3-phase  Instantaneous  Active & Reactive Power1/2
  3-phase  Instantaneous  Active & Reactive Power1/1 -> 1/sqrt(2)1/1
  1/sqrt(2)1/1 -> Demux1/1
  Demux1/2 -> Scope/2, [Q_term1]
  Demux1/1 -> Scope/1, [P_term1]
  "Excitation System "/1 -> Scope1/1, [efd]
  Multiport Switch1/1 -> Scope1/2, "Excitation System "/1
  Speed Regulator/1(Pmec) -> SM/1
  Bus Selector/2 -> [Vd]  "<Stator voltage  vd (pu)>"
  Bus Selector/3 -> [Vq]  "<Stator voltage  vq (pu)>"
  [Vq] -> "Excitation System "/3
  [Vd] -> "Excitation System "/2
  Ground/1 -> "Excitation System "/4
  connections:
  B-term/LConn3 -- SM/RConn3 -- Gen Load/LConn3
  B-term/LConn2 -- Gen Load/LConn2 -- SM/RConn2
  Gen Load/LConn1 -- B-term/LConn1 -- SM/RConn1
  B-term/RConn1 -- A/RConn1
  B-term/RConn2 -- B/RConn1
  B-term/RConn3 -- C/RConn1

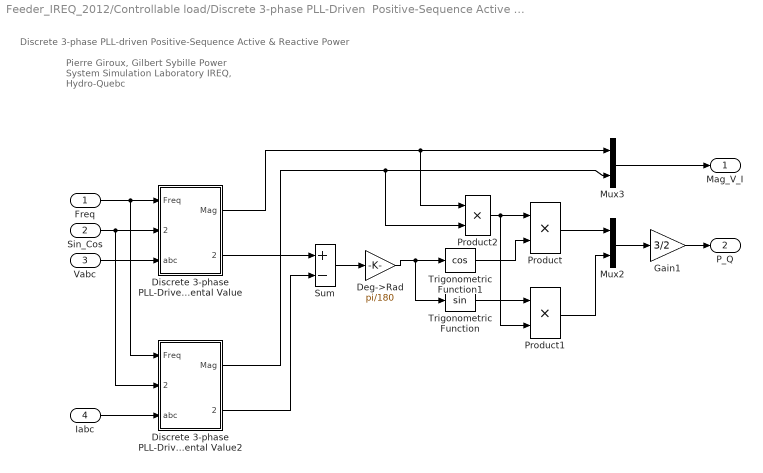
== system Feeder_IREQ_2012/Controllable load/Discrete 3-phase PLL-Driven  Positive-Sequence Active & Reactive Power ==
  note: Pierre Giroux, Gilbert Sybille
      | Power System Simulation Laboratory
      | IREQ, Hydro-Quebc
  note: Discrete 3-phase PLL-driven Positive-Sequence Active & Reactive Power
  Freq : Inport  PortDimensions=1
  Sin_Cos : Inport  Port=2  PortDimensions=2
  Vabc : Inport  Port=3  PortDimensions=3
  Iabc : Inport  Port=4  PortDimensions=3
  Deg->Rad : Gain  Gain=pi/180  SaturateOnIntegerOverflow=on  OutDataTypeStr=Inherit: Same as input  ParamDataTypeStr=Inherit: Same as input
  Discrete 3-phase PLL-Driven Positive-Sequence Fundamental Value : Subsystem  mask(Discrete 3-phase PLL-Driven Positive-Sequence Fundamental Value){Finit=Finit, Fmin=Fmin, Par_Init=Par_Vinit, Ts=Ts}
      mask prompts: Finit "Initial frequency (Hz):"; Fmin "Minimum frequency (Hz):"; Par_Init "Initial input (positive component): [ Mag  Phase-relative-to-PLL(degrees) ]"; Ts "Sample time:"
      mask help:
      | For a supplied fundamental frequency (port Freq), this discrete block computes  the positive-sequence component (Magnitude and Phase)  of a set of three balanced or unbalanced signals (port abc) which may contain harmonics.
      |  Input port "Sin_Cos" (a two-dimension signal) provides the reference frame required for the computation..
      |  First and second outputs return respectively the magnitude and phase (in degrees relative to the PLL phase)) of the fundamental.
      | For the first cycle of simulation, the outputs are held constant to the values specified by the parameter "Initial input".
      | constant to the values specified by the parameter "Initial input". The value of the parameter "Minimum frequency" is used to determine the buffer size of the "Variable Transport Delay" block found inside this subsystem.
      mask init:
      | Real_Init=Par_Init(1)*cos(pi/180*Par_Init(2));
      | Imag_Init=Par_Init(1)*sin(pi/180*Par_Init(2));
      | power_initmask();
      settings: OpenFcn=power_openblockproxy();
  Discrete 3-phase PLL-Driven Positive-Sequence Fundamental Value2 : Subsystem  mask(Discrete 3-phase PLL-Driven Positive-Sequence Fundamental Value){Finit=Finit, Fmin=Fmin, Par_Init=Par_Iinit, Ts=Ts}
      mask prompts: Finit "Initial frequency (Hz):"; Fmin "Minimum frequency (Hz):"; Par_Init "Initial input (positive component): [ Mag  Phase-relative-to-PLL(degrees) ]"; Ts "Sample time:"
      mask help:
      | For a supplied fundamental frequency (port Freq), this discrete block computes  the positive-sequence component (Magnitude and Phase)  of a set of three balanced or unbalanced signals (port abc) which may contain harmonics.
      |  Input port "Sin_Cos" (a two-dimension signal) provides the reference frame required for the computation..
      |  First and second outputs return respectively the magnitude and phase (in degrees relative to the PLL phase)) of the fundamental.
      | For the first cycle of simulation, the outputs are held constant to the values specified by the parameter "Initial input".
      | constant to the values specified by the parameter "Initial input". The value of the parameter "Minimum frequency" is used to determine the buffer size of the "Variable Transport Delay" block found inside this subsystem.
      mask init:
      | Real_Init=Par_Init(1)*cos(pi/180*Par_Init(2));
      | Imag_Init=Par_Init(1)*sin(pi/180*Par_Init(2));
      | power_initmask();
      settings: OpenFcn=power_openblockproxy();
  Gain1 : Gain  Gain=3/2  SaturateOnIntegerOverflow=on  OutDataTypeStr=Inherit: Same as input  ParamDataTypeStr=Inherit: Same as input
  Mux2 : Mux  Inputs=2
  Mux3 : Mux  Inputs=2
  Product : Product  SaturateOnIntegerOverflow=on  InputSameDT=on  OutDataTypeStr=Inherit: Same as first input
  Product1 : Product  SaturateOnIntegerOverflow=on  InputSameDT=on  OutDataTypeStr=Inherit: Same as first input
  Product2 : Product  SaturateOnIntegerOverflow=on  InputSameDT=on  OutDataTypeStr=Inherit: Same as first input
  Sum : Sum  Inputs=+-  SaturateOnIntegerOverflow=on  InputSameDT=on  OutDataTypeStr=Inherit: Same as first input
  Trigonometric Function : Trigonometry
  Trigonometric Function1 : Trigonometry  Operator=cos
  Mag_V_I : Outport
  P_Q : Outport  Port=2
  wires:
  Iabc/1 -> Discrete 3-phase PLL-Driven Positive-Sequence Fundamental Value2/3(abc)
  Discrete 3-phase PLL-Driven Positive-Sequence Fundamental Value2/1(Mag) -> Product2/2, Mux3/2
  Product2/1 -> Product1/2, Product/1
  Gain1/1 -> P_Q/1
  Mux3/1 -> Mag_V_I/1
  Product1/1 -> Mux2/2
  Product/1 -> Mux2/1
  Mux2/1 -> Gain1/1
  Trigonometric Function/1 -> Product1/1
  Trigonometric Function1/1 -> Product/2
  Deg->Rad/1 -> Trigonometric Function/1, Trigonometric Function1/1
  Sum/1 -> Deg->Rad/1
  Discrete 3-phase PLL-Driven Positive-Sequence Fundamental Value2/2(Phase) -> Sum/2
  Discrete 3-phase PLL-Driven Positive-Sequence Fundamental Value/1(Mag) -> Product2/1, Mux3/1
  Discrete 3-phase PLL-Driven Positive-Sequence Fundamental Value/2(Phase) -> Sum/1
  Sin_Cos/1 -> Discrete 3-phase PLL-Driven Positive-Sequence Fundamental Value2/2(Sin_Cos), Discrete 3-phase PLL-Driven Positive-Sequence Fundamental Value/2(Sin_Cos)
  Freq/1 -> Discrete 3-phase PLL-Driven Positive-Sequence Fundamental Value2/1(Freq), Discrete 3-phase PLL-Driven Positive-Sequence Fundamental Value/1(Freq)
  Vabc/1 -> Discrete 3-phase PLL-Driven Positive-Sequence Fundamental Value/3(abc)

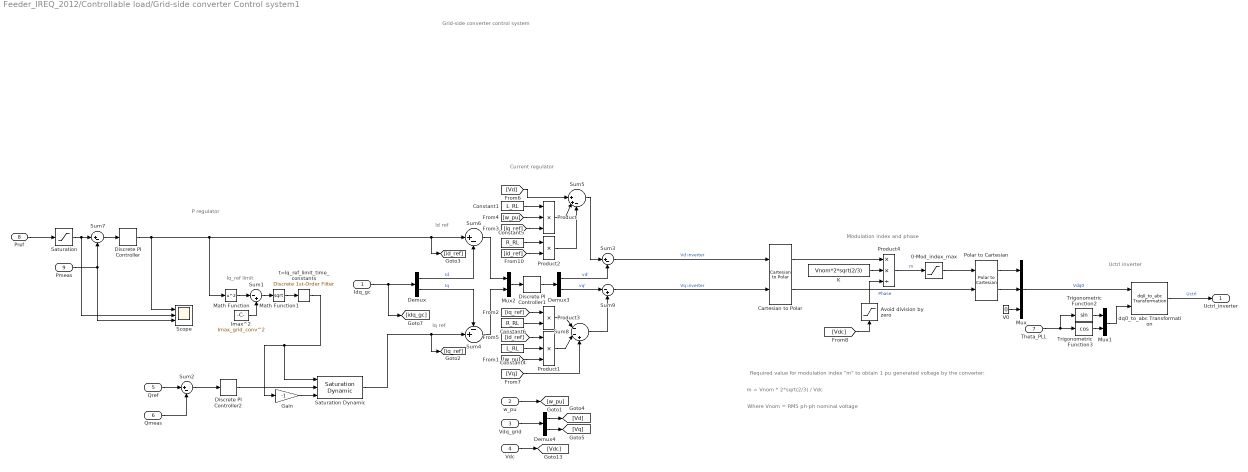
== system Feeder_IREQ_2012/Controllable load/Grid-side converter Control system1 ==
  note: Grid-side converter control system
  note: P regulator
  note: Iq_ref limit
  note: Current regulator
  note: Id ref
  note: Iq ref
  note: Required value for modulation index "m" to obtain 1 pu generated voltage by the converter:
  note: m = Vnom * 2*sqrt(2/3) / Vdc
  note: Where Vnom = RMS ph-ph nominal voltage
  note: Modulation index and phase
  note: Uctrl inverter
  Idq_gc : Inport
  w_pu : Inport  Port=2
  Vdq_grid : Inport  Port=3
  Vdc : Inport  Port=4
  Qref : Inport  Port=5
  Qmeas : Inport  Port=6
  Theta_PLL : Inport  Port=7
  Pref : Inport  Port=8
  Pmeas : Inport  Port=9
  0-Mod_index_max : Saturate  UpperLimit=Mod_index_max  LowerLimit=0
  Avoid division by zero : Saturate  UpperLimit=1e6  LowerLimit=1e-6
  Cartesian to Polar : simulink_extras/Transformations/Cartesian to Polar
  Constant1 : Constant  Value=L_RL
  Constant4 : Constant  Value=L_RL
  Constant5 : Constant  Value=R_RL
  Constant6 : Constant  Value=R_RL
  Demux : Demux  Outputs=2
  Demux3 : Demux  Outputs=2
  Demux4 : Demux  Outputs=2
  Discrete PI Controller : powerlib_extras/Discrete  Control Blocks/Discrete PI Controller  Kp=1  Ki=50  Par_Limits=[1 -1]*Imax_grid_conv  Init=0  Ts=Ts
  Discrete PI Controller1 : powerlib_extras/Discrete  Control Blocks/Discrete PI Controller  Kp=1  Ki=50  Par_Limits=[1 -1]*Current_reg_output_limit  Init=0  Ts=Ts
  Discrete PI Controller2 : powerlib_extras/Discrete  Control Blocks/Discrete PI Controller  Kp=1  Ki=50  Par_Limits=[1 -1]*Imax_grid_conv  Init=0  Ts=Ts
  Gain : Gain  Gain=-1  SaturateOnIntegerOverflow=on  OutDataTypeStr=Inherit: Same as input  ParamDataTypeStr=Inherit: Same as input
  Imax^2 : Constant  Value=Imax_grid_conv^2
  K : Constant  Value=Vnom*2*sqrt(2/3)
  Math Function : Math  Operator=square  SaturateOnIntegerOverflow=on
  Math Function1 : Math  Operator=sqrt  SaturateOnIntegerOverflow=on
  Mux : Mux  Inputs=3
  Mux1 : Mux  Inputs=2
  Mux2 : Mux  Inputs=2
  Polar to Cartesian : simulink_extras/Transformations/Polar to Cartesian
  Product : Product  Inputs=3  SaturateOnIntegerOverflow=on  InputSameDT=on  OutDataTypeStr=Inherit: Same as first input
  Product1 : Product  Inputs=3  SaturateOnIntegerOverflow=on  InputSameDT=on  OutDataTypeStr=Inherit: Same as first input
  Product2 : Product  SaturateOnIntegerOverflow=on  InputSameDT=on  OutDataTypeStr=Inherit: Same as first input
  Product3 : Product  SaturateOnIntegerOverflow=on  InputSameDT=on  OutDataTypeStr=Inherit: Same as first input
  Product4 : Product  Inputs=**/  SaturateOnIntegerOverflow=on  InputSameDT=on  OutDataTypeStr=Inherit: Same as first input
  Saturation : Saturate  UpperLimit=Pbat/Pnom  LowerLimit=0
  Saturation Dynamic : simulink/Discontinuities/Saturation Dynamic  OutMin=[]  OutMax=[]  OutDataTypeStr=Inherit: Same as second input  OutDataType=fixdt(1, 16)  OutScaling=2^-10  DoSatur=off
  Scope : Scope  NumInputPorts=3
  Sum1 : Sum  Inputs=|-+  SaturateOnIntegerOverflow=on  InputSameDT=on  OutDataTypeStr=Inherit: Same as first input
  Sum{2..3,6..7} (4 alike) : Sum  Inputs=|+-  SaturateOnIntegerOverflow=on  InputSameDT=on  OutDataTypeStr=Inherit: Same as first input
  Sum4 : Sum  Inputs=-+|  SaturateOnIntegerOverflow=on  InputSameDT=on  OutDataTypeStr=Inherit: Same as first input
  Sum5 : Sum  Inputs=||++-  SaturateOnIntegerOverflow=on  InputSameDT=on  OutDataTypeStr=Inherit: Same as first input
  Sum8 : Sum  Inputs=|--+  SaturateOnIntegerOverflow=on  InputSameDT=on  OutDataTypeStr=Inherit: Same as first input
  Sum9 : Sum  Inputs=|-+  SaturateOnIntegerOverflow=on  InputSameDT=on  OutDataTypeStr=Inherit: Same as first input
  Trigonometric Function2 : Trigonometry
  Trigonometric Function3 : Trigonometry  Operator=cos
  V0 : Constant  Value=0
  dq0_to_abc Transformation : powerlib_extras/Measurements/dq0_to_abc Transformation
  t=Iq_ref_limit_time_constants : powerlib_extras/Discrete  Control Blocks/Discrete 1st-Order Filter  FilterType=Lowpass  Tc=Iq_ref_limit_time_constant  Ts=Ts  Initialize=on  Vac_Init=[0 0 0]  Vdc_Init=Imax_grid_conv  PlotResponse=off  param1=[1 500 0.1]
  Uctrl_inverter : Outport
  wires:
  Vdc/1 -> [Vdc]
  Vdq_grid/1 -> Demux4/1
  Discrete PI Controller/1 -> Math Function/1, Sum6/1, [id_ref], Scope/1
  Qmeas/1 -> Sum2/2
  Sum2/1 -> Discrete PI Controller2/1
  Math Function1/1 -> t=Iq_ref_limit_time_constants/1
  Sum1/1 -> Math Function1/1
  Imax^2/1 -> Sum1/2
  Math Function/1 -> Sum1/1
  t=Iq_ref_limit_time_constants/1 -> Gain/1, Saturation Dynamic/1
  Constant4/1 -> Product1/2
  Discrete PI Controller1/1 -> Demux3/1
  Mux2/1 -> Discrete PI Controller1/1
  Constant1/1 -> Product/1
  Demux/2 -> Sum4/1  "Iq"
  Demux/1 -> Sum6/2  "Id"
  Product/1 -> Sum5/2
  Constant5/1 -> Product2/1
  Constant6/1 -> Product3/2
  Product1/1 -> Sum8/2
  Product2/1 -> Sum5/3
  Product3/1 -> Sum8/1
  Sum6/1 -> Mux2/1
  Sum4/1 -> Mux2/2
  [w_pu] -> Product1/3
  [w_pu] -> Product/2
  [iq_ref] -> Product/3
  [id_ref] -> Product2/2
  [iq_ref] -> Product3/1
  [id_ref] -> Product1/1
  Demux3/1 -> Sum3/2  "vd'"
  Demux3/2 -> Sum9/1  "vq'"
  w_pu/1 -> [w_pu]
  Demux4/1 -> [Vd]
  Demux4/2 -> [Vq]
  [Vq] -> Sum8/3
  [Vd] -> Sum5/1
  Product4/1 -> 0-Mod_index_max/1  "m"
  K/1 -> Product4/2
  Avoid division by zero/1 -> Product4/3
  Cartesian to Polar/1 -> Product4/1
  [Vdc] -> Avoid division by zero/1
  Polar to Cartesian/2 -> Mux/2
  Polar to Cartesian/1 -> Mux/1
  V0/1 -> Mux/3
  Trigonometric Function3/1 -> Mux1/2
  Trigonometric Function2/1 -> Mux1/1
  Mux1/1 -> dq0_to_abc Transformation/2
  Cartesian to Polar/2 -> Polar to Cartesian/2  "Phase"
  Mux/1 -> dq0_to_abc Transformation/1  "Vdq0"
  dq0_to_abc Transformation/1 -> Uctrl_inverter/1  "Uctrl"
  Idq_gc/1 -> [idq_gc], Demux/1
  0-Mod_index_max/1 -> Polar to Cartesian/1
  Sum5/1 -> Sum3/1
  Sum8/1 -> Sum9/2
  Pref/1 -> Saturation/1
  Qref/1 -> Sum2/1
  Gain/1 -> Saturation Dynamic/3
  Discrete PI Controller2/1 -> Saturation Dynamic/2
  Pmeas/1 -> Sum7/2, Scope/3
  Saturation Dynamic/1 -> Sum4/2, [iq_ref]
  Saturation/1 -> Scope/2, Sum7/1
  Sum7/1 -> Discrete PI Controller/1
  Theta_PLL/1 -> Trigonometric Function2/1, Trigonometric Function3/1
  Sum3/1 -> Cartesian to Polar/1  "Vd inverter"
  Sum9/1 -> Cartesian to Polar/2  "Vq inverter"

== system Feeder_IREQ_2012/Diesel Generator/Reactive power gain1 ==
  In1 : Inport
  Product : Product  RndMeth=Zero
  Product1 : Product  RndMeth=Zero
  Sign : Signum
  Trigonometric Function1 : Trigonometry  Operator=acos
  Trigonometric Function2 : Trigonometry  Operator=tan
  Out1 : Outport
  wires:
  In1/1 -> Sign/1, Product/2
  Sign/1 -> Product/1, Product1/1
  Product/1 -> Trigonometric Function1/1
  Trigonometric Function1/1 -> Product1/2
  Product1/1 -> Trigonometric Function2/1
  Trigonometric Function2/1 -> Out1/1
